simulink library "commsink"  (Simulink 5.0)
values from neighbouring files (symbols this model uses):
  ts = td(1)    [commblkreadwkspc.m]    (also in eyesampl.m = [sampleTime(1), sampleTime(2)])
undefined symbols (not defined in the file or in its folder): eyediasi, eyesampl, td
settings Model: RequirementInfo=9  Creator=tdelve  LastModifiedBy=mmclerno

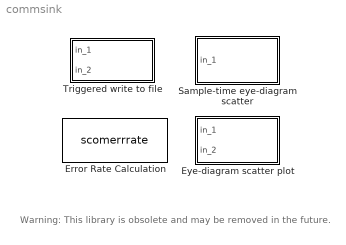
== system commsink ==
  note: Warning:  This library is obsolete and may be
      | removed in the future.
  Error Rate Calculation : S-Function  FunctionName=scomerrrate  Parameters=N, st_delay, cp_mode, subframe, PMode, WsName, RsMode2  mask(Error Rate Calculation){N=0, st_delay=0, cp_mode=Entire frame, subframe=[], PMode=Workspace, WsName=ErrorVec, RsMode2=off}
      mask prompts: N "Receive delay:"; st_delay "Computation delay:"; cp_mode "Computation mode:"; subframe "Selected samples from frame:"; PMode "Output data:"; WsName "Variable name:"; RsMode2 "Reset port"
      mask help:
      | Compute the error rate of the received data by comparing it to a delayed version of the transmitted data.  The delays are specified in number of samples, regardless of whether the input is a scalar or vector.
      |
      | The 'Computation mode' parameter allows the block to compare only certain portions of each frame.  For example, to compare only the first 10 and last 6 values in a frame of 80 symbols, set 'Computation mode' to 'Select samples from mask' and set 'Selected samples from frame' to [1:10 75:80].
      |
      | The block output is a three-element vector consisting of the error rate, followed by the number of errors detected and the total number of symbols compared.  This vector can be sent to either the workspace or an output port.
      mask init:
      | [s] = commblkerrrate(gcb,'init');
      | if(PMode==1)
      |     if(isempty(WsName))
      |         error('Output variable name cannot be empty.')
      |     end
      |     if(~isletter(WsName(1)))
      |         error('Output variable name must be a string.')
      |     end
      | end
      mask StyleString: edit,edit,popup(Entire frame|Select samples from mask|Select samples from port),edit,popup(Workspace|Port),edit,checkbox
      mask CallbackString: ||commblkerrrate(gcb,'CpMode');||commblkerrrate(gcb,'OutMode');||
      mask Display:
      | disp('Error Rate\nCalculation');
      | port_label('input',s.i1,s.i1s);
      | port_label('input',s.i2,s.i2s);
      | port_label('input',s.i3,s.i3s);
      | port_label('input',s.i4,s.i4s);
  Eye-diagram scatter plot : Subsystem  LoadFcn=eyediasi([],[],[],'LoadBlock')  StartFcn=eyediasi([],[],[],'Start')  StopFcn=eyediasi([],[],[],'Stop')  mask(Eye-diagram/scatter plot){time_range=.2, boundary=[-1.5 1.5], kept_length=5, eye_line='y-/r-', scatter_line='y./g*', two_d_line='g-/y-.'}
      mask prompts: time_range "Eye-pattern plot time frame:"; boundary "Lower and upper bound of in-coming signal (1x2 vector):"; kept_length "Number of saved traces:"; eye_line "Line-type for eye-pattern diagram (0 for no plot):"; scatter_line "Line-type for scatter plot (0 for no plot):"; two_d_line "Line-type for x-y plot (0 for no plot):"
      mask help: Produce eye-pattern diagram/scatter plot/x-y plot with the rising edge of the second input as the decision line.
      mask init:
      | [x,y]=trigicon(0,25,get_param(gcb,'orientation'),2);
      settings: CopyFcn=eyediasi([],[],[],'CopyBlock')  DeleteFcn=eyediasi([],[],[],'DeleteBlock')  NameChangeFcn=eyediasi([],[],[],'NameChange')
      mask Help: This plot opens one, two, or three plots by assigning the line type parameters. The scatter plot point is selected by the rising edge of a trigger signal. A decision line is drawn at the rising edge of the trigger signal.
      mask Display: plot(0,0,100,100,[5 95 95 5 5 5 5+90*[0:1/30:1] 5+90*[1:-1/30:0]],[35 35 95 95 35 65 sin([0:1/30:1]*pi*2)*25+65 sin([0:1/30:1]*pi*2)*25+65]*.8+9, x,y);
  Sample-time eye-diagram scatter : Subsystem  LoadFcn=eyesampl([],[],[],'LoadBlock')  StartFcn=eyesampl([],[],[],'Start')  StopFcn=eyesampl([],[],[],'Stop')  mask(Eye-diagram/scatter plot){time_range=[td, .05 .1], boundary=[-1.5 1.5], kept_length=5, eye_line='y-/r-', scatter_line='y./g*', two_d_line=ts}
      mask prompts: time_range "[Symbol interval, plot offset, decision point offset]:"; boundary "Lower and upper bound of in-coming signal (1x2 vector):"; kept_length "Number of saved traces:"; eye_line "Line-type for eye-pattern diagram (0 for no plot):"; scatter_line "Line-type for scatter plot (0 for no plot):"; two_d_line "Plot update sample time:"
      mask help: Produce eye-pattern diagram and/or scatter plot.
      settings: CopyFcn=eyesampl([],[],[],'CopyBlock')  DeleteFcn=eyesampl([],[],[],'DeleteBlock')  NameChangeFcn=eyesampl([],[],[],'NameChange')
      mask Help: This plot opens one, or two plots by assigning the line type parameters. The scatter plot point is selected by the decision point in the first parameter entry. A decision line is drawn in the eye-pattern diagram. The plot is updated at the plot update sample time point.
      mask Display: plot(0,0,100,100,[5 95 95 5 5 5 5+90*[0:1/30:1] 5+90*[1:-1/30:0]],[35 35 95 95 35 65 sin([0:1/30:1]*pi*2)*25+65 sin([0:1/30:1]*pi*2)*25+65]);
  Triggered write to file : Subsystem  mask(Write to file){filename='junk.dat', datatype='ascii', nump=0, threshold=0.5}
      mask prompts: filename "File name (string, include extension):"; datatype "Data type ('ascii', 'float', 'integer'):"; nump "Number of trigger pulses between saved data:"; threshold "Threshold in detecting trigger signal:"
      mask help: The rising edge of the signal from the 2nd port triggers the block to write another row into the specified file.
      mask init:
      | [x,y]=trigicon(0,25,get_param(gcb,'orientation'),2);
      mask Help: This block writes the data input from the first port to the next row of the specified file at the rising edge of the second input trigger pulse. The first pulse triggers to write the first record. You can specify the number of pulses between writting records. When you specify ASCII format, there is no return added between two records.
      mask Display:
      | plot(0,0,100,100,100-[25 25 05 05 25 25 05 13 13 17 17 17 15 real(exp(j*pi*([0:20]/10+1/2)))*3.5+15 15 25 25 25+[0:1/30:1]*70],
      | [85 95 95 75 75 89 89 89 95 95 89 89 89 imag(exp(j*pi*([0:20]/10+1/2)))*3.5+85 89 89 85 -sin([0:1/30:1]*pi*2)*10+85]-15, x,y);disp('\nWt file')

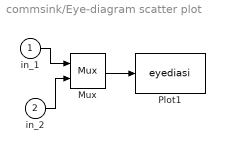
== system commsink/Eye-diagram scatter plot ==
  in_1 : Inport
  in_2 : Inport  Port=2
  Mux : Mux  Inputs=2
  Plot1 : S-Function  FunctionName=eyediasi  Parameters=time_range, boundary, kept_length, eye_line, scatter_line, two_d_line
  wires:
  Mux/1 -> Plot1/1
  in_2/1 -> Mux/2
  in_1/1 -> Mux/1

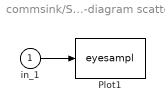
== system commsink/Sample-time eye-diagram scatter ==
  in_1 : Inport
  Plot1 : S-Function  FunctionName=eyesampl  Parameters=time_range, boundary, kept_length, eye_line, scatter_line, two_d_line
  wires:
  in_1/1 -> Plot1/1

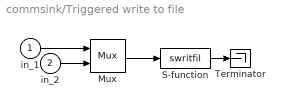
== system commsink/Triggered write to file ==
  in_1 : Inport
  in_2 : Inport  Port=2
  Mux : Mux  Inputs=2
  S-function : S-Function  FunctionName=swritfil  Parameters=filename, datatype, nump, threshold
  Terminator : Terminator
  wires:
  in_2/1 -> Mux/2
  in_1/1 -> Mux/1
  Mux/1 -> S-function/1
  S-function/1 -> Terminator/1
